simulink model "Lab_Delay_Abs_Sign_PWM"  (R2024b)
settings: Solver=VariableStepAuto  StartTime=0.0  StopTime=10.0  RelTol=1e-3
libraries: simulink x1
settings Model: Creator=Ahmad  LastModifiedBy=Ahmad

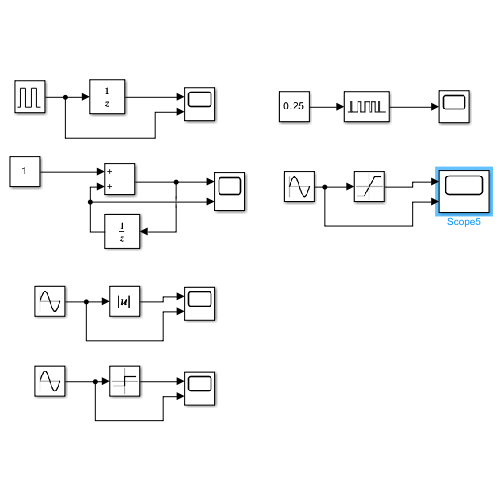
[thumbnail: Simulink's stored preview of the top-level diagram]
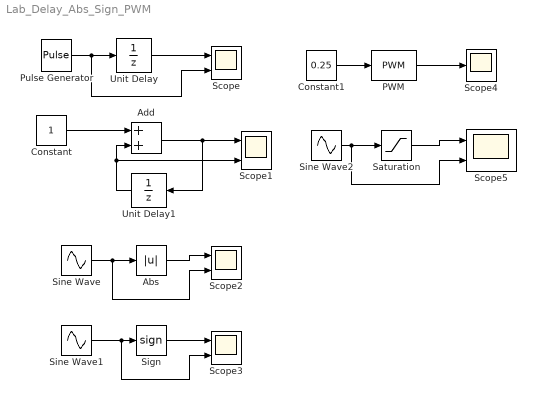
== system Lab_Delay_Abs_Sign_PWM ==
  Abs : Abs  SaturateOnIntegerOverflow=off
  Add : Sum
  Constant : Constant
  Constant1 : Constant  Value=0.25
  PWM : simulink/Discontinuities/PWM  DisableCoverage=on  Period=1  InitialDelay=0  DisallowZeroDutyCycle=off  RunAtFixedTimeIntervals=off  SampleTime=0.1
  Pulse Generator : DiscretePulseGenerator  PulseType=Time based  Period=1  PulseWidth=25
  Saturation : Saturate
  Scope{,1..3,5} (5 alike) : Scope  NumInputPorts=2
  Scope4 : Scope
  Sign : Signum
  Sine Wave : Sin  SampleTime=0
  Sine Wave1 : Sin  SampleTime=0
  Sine Wave2 : Sin  SampleTime=0
  Unit Delay : UnitDelay  SampleTime=-1  HasFrameUpgradeWarning=on
  Unit Delay1 : UnitDelay  SampleTime=-1  HasFrameUpgradeWarning=on
  wires:
  Pulse Generator/1 -> Scope/2, Unit Delay/1
  Unit Delay/1 -> Scope/1
  Constant/1 -> Add/1
  Add/1 -> Scope1/1, Unit Delay1/1
  Unit Delay1/1 -> Scope1/2, Add/2
  Abs/1 -> Scope2/1
  Sine Wave/1 -> Scope2/2, Abs/1
  Sine Wave1/1 -> Scope3/2, Sign/1
  Sign/1 -> Scope3/1
  Constant1/1 -> PWM/1
  PWM/1 -> Scope4/1
  Sine Wave2/1 -> Scope5/2, Saturation/1
  Saturation/1 -> Scope5/1
